simulink model "p_i"  (R2019b)
settings: Solver=VariableStepAuto  StartTime=0.0  StopTime=10.0  RelTol=1e-3
InitFcn:
  | PM = 75
  | 
  | Wc = 20
  | 
  | pi = tand(PM - 90 + atand((Wc*0.0015806)/0.0034));
  | 
  | Ki= (Wc * sqrt(0.0034^2 + (Wc*0.0015806)^2))/sqrt(1+(pi)^2);
  | 
  | Kp= (pi*Ki)/Wc;
settings Model: OrderedModelArguments=off  Creator=kanth  LastModifiedBy=kanth

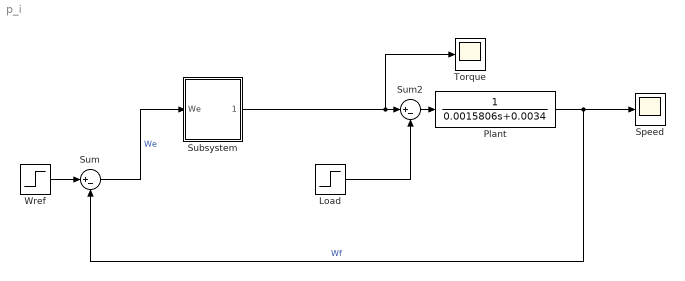
== system p_i ==
  Load : Step  Time=5  After=5  SampleTime=0
  Plant : TransferFcn  Denominator=[0.0015806 0.0034]
  Speed : Scope
  Subsystem : Subsystem
  Sum : Sum  Inputs=|+-
  Sum2 : Sum  Inputs=|+-
  "Torque " : Scope
  Wref : Step  After=1400  SampleTime=0
  wires:
  Plant/1 -> Speed/1, Sum/2  "Wf"
  Wref/1 -> Sum/1
  Load/1 -> Sum2/2
  Sum2/1 -> Plant/1
  Subsystem/1(Torque) -> "Torque "/1, Sum2/1
  Sum/1 -> Subsystem/1(We)  "We"

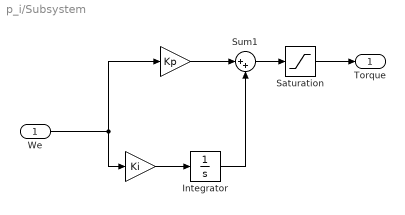
== system p_i/Subsystem ==
  We : Inport
  " " : Gain  Gain=Kp
  "  " : Gain  Gain=Ki
  Integrator : Integrator  LimitOutput=on  UpperSaturationLimit=10  LowerSaturationLimit=-10
  Saturation : Saturate  UpperLimit=12  LowerLimit=-12
  Sum1 : Sum  Inputs=|++
  Torque : Outport
  wires:
  Saturation/1 -> Torque/1
  "  "/1 -> Integrator/1
  Integrator/1 -> Sum1/2
  We/1 -> "  "/1, " "/1
  " "/1 -> Sum1/1
  Sum1/1 -> Saturation/1
